simulink model "TestHz"  (R2020b)
settings: Solver=FixedStepDiscrete  StartTime=0.0  StopTime=inf  FixedStep=Ts  RelTol=1e-3
values from neighbouring files (symbols this model uses):
  g = 9.81    [equpoint.m]    (also in plotAMS.m; plotAMS2.m)
  J = diag([0.0056 0.0056 0.0104])    [equpoint.m]
  m = 0.7    [equpoint.m]    (also in plotAMS.m = 0.752; plotAMS2.m = 0.752)
  M = ([ 1          1          1         1 ... (first row only)    [allocation.m]    (also in equpoint.m; plotAMS.m; plotAMS2.m)
undefined symbols (not defined in the file or in its folder): B, MY_ATT_P, MY_ATT_P_YAW, MY_POS_P, MY_RATE_P, MY_RATE_P_YAW, MY_SAT_AD, MY_TAU_P_A, MY_TAU_P_A_YAW, MY_TAU_P_P, MY_TAU_P_P_YAW, MY_VEL_P, T00, Tf, Tmotorbar, Ts
libraries: discretizing x10, pixhawk_slib_uORB_RW x6, pixhawk_slib_sensors_actuators x5, pixhawk_slib_misc_utils x1, simulink x1, sharedtransform x1, pid_lib x1
(part 2 of 2)

== matlab function TestHz/controller/innerloop/MATLAB Function1 ==
  data: u input; y output
function y = fcn(u)
y=diag([u,1,1,1]);

== matlab function TestHz/controller/innerloop/MATLAB Function2 ==
  data: dT input; ub output
function ub = fcn(dT)
dub = zeros(4,1);
dub(1) = dT(1) - dT(3);
dub(2) = dT(2) - dT(4);
dub(3) = dT(3) - dT(1);
dub(4) = dT(4) - dT(2);
% dub(1) = dT(1);
% dub(2) = dT(2);
% dub(3) = dT(3);
% dub(4) = dT(4);
ub = [5 5 5 5]' + 1.8*min([dub(1) dub(2) dub(3) dub(4)]',[0 0 0 0]');%1.8

== matlab function TestHz/controller/InputConditioning/MATLAB Function ==
  data: u input; y output
function y = fcn(u)

 if(u>1550)
    y=u;
 else
     if(u<1450)
     y=u;
     else
         y=single(1500);
     end
 end

== matlab function TestHz/controller/InputConditioning/MATLAB Function1 ==
  data: u input; y output
function y = fcn(u)

 if(u>1550)
    y=u;
 else
     if(u<1450)
     y=u;
     else
         y=single(1500);
     end
 end

== matlab function TestHz/controller/InputConditioning/MATLAB Function2 ==
  data: u input; y output
function y = fcn(u)

 if(u>1550)
    y=u;
 else
     if(u<1450)
     y=u;
     else
         y=single(1500);
     end
 end

== matlab function TestHz/controller/quat2eul ==
  data: q input single; dcm output single
function dcm  = quat2eul(q)
% Conversion from Quaternion to Euler angles based on the PX4 Firmware
% v1.6.5 release.
% 
% Quaternion -> DCM -> Euler Angles
% INPUT:
%   q: Quaternion vector of the format: (a + bi + cj + dk)
% OUTPUT:
%   [phi,theta,psi]: Euler angles in radians.
% 
 if norm(q)~=0
    a = q(1);
    b = q(2);
    c = q(3);
    d = q(4);

    aSq = a*a;
    bSq = b*b;
    cSq = c*c;
    dSq = d*d;

    d_pi2 = pi/2;

    % quaternion_to_dcm
    dcm00 = aSq + bSq - cSq - dSq;
    dcm01 = 2*(b*c - a*d);
    dcm02 = 2*(a*c + b*d);
    dcm10 = 2*(b*c + a*d);
    dcm11 = aSq - bSq + cSq - dSq;
    dcm12 = 2*(c*d - a*b);
    dcm20 = 2*(b*d - a*c);
    dcm21 = 2*(a*b + c*d);
    dcm22 = aSq - bSq - cSq + dSq;
    dcm=[dcm00 dcm01 dcm02;
              dcm10 dcm11 dcm12;
              dcm20 dcm21  dcm22];
 else
     dcm = single(eye(3,3));
 end
    % dcm_to_euler

== matlab function TestHz/controller/innerloop/Att ==
  data: e input; w input; psi input; pqrd output; ATT_P input; ATT_P_SCALE input
function pqrd  = fcn(e, w, psi, ATT_P, ATT_P_SCALE)
%% 角度控制1
% h1 = n3(1);
% h2 = n3(2);
% h3 = n3(3);
% h1d = n3d(1);
% h2d = n3d(2);
% h3d = n3d(3);
% we = Reb*w;
% k1 = single(5);
% epqd = [0 -1/h3; 1/h3 0]*[k1*(h1d-h1)+h2*we(3);k1*(h2d-h2)-h1*we(3)];
% 
% psid = single(0);
% rd = k1*0.3*(psid - psi);
% 
% Rbe = Reb';
% erd = (rd - Rbe(3,1)*epqd(1) - Rbe(3,2)*epqd(2))/Rbe(3,3);
% 
% pqd = Rbe((1:2),:)*[epqd; erd];%计算出机体系下的pqd
% pqd = mysat(pqd,2);
% pqrd = [pqd;rd];
%% 角度控制2
e1 = e(1);
e2 = e(2);
% e1  = n3(1) - n3d(1);
% e2  = n3(2) - n3d(2); 
beta = atan2(e2,e1);

k1 = ATT_P;
pqd = [ -k1*sqrt(e1^2+e2^2)*sin(psi-beta);
             -k1*sqrt(e1^2+e2^2)*cos(psi-beta);];
pqd = mysatsingle(pqd,3);
psid = 0;
% rd = -k1*0.3*(psi-psid);
rd = -k1*ATT_P_SCALE*(psi-psid);
% rd = 0;
pqrd = [pqd;rd];

== matlab function TestHz/controller/Subsystem1/d_z ==
  data: n3 input size=[3,1]; dvz input single size=1; T_ input single size=4; M input single size=[4,4]; m input single size=1; g input single size=1; dz output single size=1
function dz   = fcn(n3, dvz, T_, M, m, g)
dz  = m*(dvz-g)/n3(3)+M(1,:)*T_;

== matlab function TestHz/controller/Subsystem1/MATLAB Function2 ==
  data: throtte input; ad output; p input; v input; vhd input; POS_P input; VEL_P input
function ad = fcn(throtte, p, v, vhd, POS_P, VEL_P)
persistent pd
if isempty(pd)
    pd = single(p);
end
%% 高度通道
if throtte>=0.4&& throtte <=0.6
        vd3 = mysatsingle(POS_P * (pd(3) - p(3)), 0.5);
        ad3 = VEL_P * (vd3 - v(3));
else
    if throtte>0.6
        vd3 = -1;
        ad3 = VEL_P * (vd3 - v(3));
        pd(3) = p(3);
    else
        vd3 = 1;
        ad3 = VEL_P * (vd3 - v(3));
        pd(3) = p(3);
    end
end
%% 水平通道
if norm(vhd) <= 0.05
        vd12 = mysatsingle(POS_P * (pd(1:2) - p(1:2)), 0.5);
        ad12 = VEL_P * (vd12 - v(1:2));
else
        vd12 = mysatsingle(5*vhd, 0.7);
        ad12 = VEL_P * (vd12 - v(1:2));
        pd(1:2) = p(1:2);
end
ad = [ad12;ad3];

== matlab function TestHz/controller/Subsystem2/MATLAB Function ==
  data: Reb input; psi output
function psi = fcn(Reb)
psi = atan2(Reb(2,1), Reb(1,1));

== matlab function TestHz/controller/Subsystem1/Pos ==
  data: ad3 input single size=[3,1]; n3 input; m input single size=1; fd output single size=1; g input single size=1; n3d output single size=3; ad output single size=3; SAT_AD input
function [fd, n3d, ad]  = fcn(ad3, n3, m, g, SAT_AD)
 

% ad3 = [ad1(1)+ad2(1); ad1(2)+ad2(2); ad1(3)+ad2(3)];

ad = mysatsingle(ad3,single(SAT_AD)*g);

n3d = ([single(0); single(0); g]-ad)/norm([single(0); single(0); g]-ad);
if n3d(3)==single(0)
    fd = single(0);
else
    fd = m*(g-ad(3))/n3(3);
%     fd = m*g-ad(3);
end
